simulink model "Rod_end_v7c"  (R2023a)
settings: Solver=ode1be  StartTime=0.0  StopTime=3  FixedStep=1e-6  MaxStep=1e-5  RelTol=1e-3
values from neighbouring files (symbols this model uses):
  A1_la = 5.710000e-003    (= 0.00571)    [C1_Actuator_1_Data.m]
  A2_la = 5.710000e-003    (= 0.00571)    [C1_Actuator_1_Data.m]
  a_jetpipe_area = 0    [B2_Main_file_Double_Active_Standby_System.m]
  A_svfb = 79.12.*1E-9.*sqrt(pi)    [B2_Main_file_Double_Active_Standby_System.m]
  a_svfb0_1 = 1E-3    (= 0.001)    [B2_Main_file_Double_Active_Standby_System.m]
  a_svfb0_2 = 0    [B2_Main_file_Double_Active_Standby_System.m]
  Afl_sv = dfl_sv^2*pi/4    (= 2.01519637574e-09)    [C1_Actuator_1_Data.m]
  Ag_sv = 18e-6    (= 1.8e-05)    [C1_Actuator_1_Data.m]
  air_gap0_1 = 0    [B2_Main_file_Double_Active_Standby_System.m]
  air_gap_fault_time = 10000    [B2_Main_file_Double_Active_Standby_System.m]
  Alpha_p0 = eta-acos((L^2+t^2-s^2)/(2*L*t))    [Parametri_rod_end.m]
  Asp_sv = 1.35e-5    (= 1.35e-05)    [C1_Actuator_1_Data.m]
  B0_sv = 0.460    (= 0.46)    [C1_Actuator_1_Data.m]
  b_airgap = 0.3    [B2_Main_file_Double_Active_Standby_System.m]
  b_fbspring = 2E-3    (= 0.002)    [B2_Main_file_Double_Active_Standby_System.m]
  b_max = 0*0.0001    (= 0)    [C1_Actuator_1_Data.m]
  beta = 800000000    [D4_Fluid.m]    (also in Rapporto_di_trasmissione.m = acos((L-t.*cos(alpha))./s))
  Beta0 = acos((L-t*cos(Alpha0))/s)    [Parametri_rod_end.m]
  beta_LVDT = 0    [aggiunte.m]
  bf_sv = 0.45    [C1_Actuator_1_Data.m]
  bsp_sv = 0.25    [C1_Actuator_1_Data.m]
  c = 55    [Parametri_rod_end.m]
  C_svfb = 1    [B2_Main_file_Double_Active_Standby_System.m]
  Cdmax_sv = 0.7392    [C1_Actuator_1_Data.m]
  Cdmin_sv = 0.6428    [C1_Actuator_1_Data.m]
  CLa = 900000    [aggiunte.m]
  Csa_la = 0.02*sqrt(Ksa_la*Meq_la)    [C1_Actuator_1_Data.m]
  Damping = 1e3    (= 1000)    [Parametri_rod_end.m]
  Damping_rot = 100    [Parametri_rod_end.m]
  Del_on = 1    [B2_Main_file_Double_Active_Standby_System.m]
  demag0_1 = 0    [B2_Main_file_Double_Active_Standby_System.m]
  dfl_sv = 5.0654e-5    (= 5.0654e-05)    [C1_Actuator_1_Data.m]
  dt_sim = 1e-5    (= 1e-05)    [B2_Main_file_Double_Active_Standby_System.m]
  enable_jetpipe_distorsion = 0    [B2_Main_file_Double_Active_Standby_System.m]
  eta = deg2rad(15)    [Parametri_rod_end.m]
  F_att_sv = 4    [C1_Actuator_1_Data.m]
  FH = FH+0.175*pi*Dd_se(ii)*(-0.884+0.0206*Hs_se(ii)-0.0001*(Hs_se(ii))^2)*Tw_se(ii)    [D2_Data_seal.m]
  first_cycle = 0    [B2_Main_file_Double_Active_Standby_System.m]
  flight_hours = 8    [B2_Main_file_Double_Active_Standby_System.m]
  g = 9.81    [Parametri_rod_end.m]
  g_sv = G_sv/l0_sv    (= 0)    [C1_Actuator_1_Data.m]
  Gamma_la = 1.667e4    (= 16670)    [C1_Actuator_1_Data.m]
  gap_ms = 0    [C1_Actuator_1_Data.m]
  Gq_sv = 0.069    [C1_Actuator_1_Data.m]
  Gust_stiffness_jetpipe = 1e8    (= 100000000)    [B2_Main_file_Double_Active_Standby_System.m]
  Gust_threshold = 10000    [B2_Main_file_Double_Active_Standby_System.m]
  h_fbspring = 1E-3    (= 0.001)    [B2_Main_file_Double_Active_Standby_System.m]
  h_sv = H_sv/l0_sv    (= 0)    [C1_Actuator_1_Data.m]
  hr_sv = 6e-6    (= 6e-06)    [C1_Actuator_1_Data.m]
  hyd_fluid_repl = 20    [B2_Main_file_Double_Active_Standby_System.m]
  I = 2.3    [Parametri_rod_end.m]    (also in Rapporto_di_trasmissione.m)
  imax_sv = 8e-3    (= 0.008)    [C1_Actuator_1_Data.m]
  Initial_condition = [0;0;0.000]    [Parametri_rod_end.m]
  Ixx_out = 0.0000321    (= 3.21e-05)    [Parametri_rod_end.m]
  Iyy_in = 0.0000008    (= 8e-07)    [Parametri_rod_end.m]
  Iyy_out = 0.0000035    (= 3.5e-06)    [Parametri_rod_end.m]
  Izz_in = 0.00000011    (= 1.1e-07)    [Parametri_rod_end.m]
  Izz_out = 0.0000337    (= 3.37e-05)    [Parametri_rod_end.m]
  Ja_sv = 1.0575e-5    (= 1.0575e-05)    [C1_Actuator_1_Data.m]
  jetpipe_initialpos = 0    [B2_Main_file_Double_Active_Standby_System.m]
  jetpipe_passage_area = 1    [B2_Main_file_Double_Active_Standby_System.m]
  k = 4/(3*pi*(sigma_j+sigma_k))*((R_in*R_out)/(R_in+R_out))^0.5    (= 15092124693.8)    [Parametri_rod_end.m]
  k_airgap = 0.5/100*0.01    (= 5e-05)    [B2_Main_file_Double_Active_Standby_System.m]
  k_c0_jetpipe_area = 0*1e-1    (= 0)    [B2_Main_file_Double_Active_Standby_System.m]
  k_sv = mup_sv*Vp_sv/(2*B0_sv*l0_sv)-1    (= 16.0383594613)    [C1_Actuator_1_Data.m]
  Kf_sv = 301.6    [C1_Actuator_1_Data.m]
  KFPi = zeros(m,1)    [D2_Data_seal.m]
  Kli1 = 0    [C1_Actuator_1_Data.m]
  Kli2 = 0    [C1_Actuator_1_Data.m]
  Ksa_la = 12480000    [C1_Actuator_1_Data.m]
  Kw_sv = 14.5    [C1_Actuator_1_Data.m]
  L = 0.37    [Parametri_rod_end.m]    (also in Rapporto_di_trasmissione.m = l+delta_l)
  l0_sv = 0.5e-3    (= 0.0005)    [C1_Actuator_1_Data.m]
  L_c = imax_sv    (= 0.008)    [C1_Actuator_1_Data.m]
  L_la1 = 0.059900    (= 0.0599)    [C1_Actuator_1_Data.m]
  L_la2 = 0.084800    (= 0.0848)    [C1_Actuator_1_Data.m]
  la_sv = 41e-3    (= 0.041)    [C1_Actuator_1_Data.m]
  lambda_LVDT = 0*0.005*1.5    (= 0)    [aggiunte.m]
  lf = 0.025    [C1_Actuator_1_Data.m]    (also in C2_Actuator_2_Data.m)
  LVDTsize0 = 1    [aggiunte.m]
  m_in = 0.0215    [Parametri_rod_end.m]
  m_out = 0.1    [Parametri_rod_end.m]
  m_thermal = 0    [B2_Main_file_Double_Active_Standby_System.m]
  Mcyl_la = 30.425550    (= 30.42555)    [C1_Actuator_1_Data.m]
  Mrod_la = 11.313490    (= 11.31349)    [C1_Actuator_1_Data.m]
  msp_sv = 0.005    [C1_Actuator_1_Data.m]
  mua_sv = 4*pi/1e7    (= 1.25663706144e-06)    [C1_Actuator_1_Data.m]
  mup_sv = 1.1*4*pi/1e7    (= 1.38230076758e-06)    [C1_Actuator_1_Data.m]
  n1_sv = 1140    [C1_Actuator_1_Data.m]
  n2_sv = 1140    [C1_Actuator_1_Data.m]
  n_svfb = 3    [B2_Main_file_Double_Active_Standby_System.m]
  null_shift = -1+2*rand(1,1)    [B2_Main_file_Double_Active_Standby_System.m]
  null_shift_sign = -1+((-1+2*rand(1,1))>=0)*2    [B2_Main_file_Double_Active_Standby_System.m]
  OV_R1 = 0*2.344e-05    (= 0)    [C1_Actuator_1_Data.m]
  OV_R2 = 0*2.344e-05    (= 0)    [C1_Actuator_1_Data.m]
  OV_S1 = 0*2.344e-05    (= 0)    [C1_Actuator_1_Data.m]
  OV_S2 = 0*2.344e-05    (= 0)    [C1_Actuator_1_Data.m]
  P01_la = Pmean-DP_eq    [C1_Actuator_1_Data.m]
  P02_la = Pmean+DP_eq    [C1_Actuator_1_Data.m]
  perc_passage_area0_1 = 0    [B2_Main_file_Double_Active_Standby_System.m]
  Pocl_A = 0    [C1_Actuator_1_Data.m]
  Pocl_B = 0    [C1_Actuator_1_Data.m]
  Pr = 600000    [B2_Main_file_Double_Active_Standby_System.m]
  Ps = 35000000    [B2_Main_file_Double_Active_Standby_System.m]
  R_in = 0.019    [Parametri_rod_end.m]
  R_out = 0.0195    [Parametri_rod_end.m]
  R_th1 = 0    [B2_Main_file_Double_Active_Standby_System.m]
  Remax_sv = 5000    [C1_Actuator_1_Data.m]
  Resistance = 1    [C1_Actuator_1_Data.m]
  rj_sv = 1e-6    (= 1e-06)    [C1_Actuator_1_Data.m]
  Rp02_svspring = 1014    [B2_Main_file_Double_Active_Standby_System.m]
  s = 0.11    [Parametri_rod_end.m]    (also in Rapporto_di_trasmissione.m)
  sigma_0LVDT = 0*0.01*1.5*5    (= 0)    [aggiunte.m]
  ST_AD = ceil(10000/fs_AD)/10000    [C1_Actuator_1_Data.m]
  Stiffness_rot = 1e3    (= 1000)    [Parametri_rod_end.m]
  Stifness = 1e8    (= 100000000)    [Parametri_rod_end.m]
  sv_crackON1 = 0    [B2_Main_file_Double_Active_Standby_System.m]
  sv_crackON2 = 0    [B2_Main_file_Double_Active_Standby_System.m]
  T0 = 0    [aggiunte.m]
  tau_w1 = 0    [B2_Main_file_Double_Active_Standby_System.m]
  ... (+14 more)
undefined symbols (not defined in the file or in its folder): Ixx_in, magnitude, mass, muu, Newton, R_sp_C, Raphson
libraries: simulink x16, matrix_library x12, sharedutil x2
(part 4 of 4)

== system Rod_end_v7c/Attuatore/Actuation System/Servovalve/Spool/orifice2S-resistences/Cd ==
  In2 : Inport
  In1 : Inport  Port=2
  In3 : Inport  Port=3
  Abs : Abs  SaturateOnIntegerOverflow=off
  Fcn : Fcn  Expr=0.22*sqrt(log(1+u(1)))
  Fcn1 : Fcn  Expr=u(2)*(1+0.2*hr_sv/(u(1)+hr_sv))
  Fcn2 : Fcn  Expr=2*u(3)*u(2)/(u(4)*(wsp_sv+u(1)))
  Fcn3 : Fcn  Expr=(u(2)*(u(1)+u(3)))/(2*(u(1)*u(3)))
  Lookup Table1 : Lookup  InputValues=R_sp_C(1,:)  Table=R_sp_C(2,:)  SaturateOnIntegerOverflow=off
  Memory1 : Memory  InitialCondition=eps
  Mux1 : Mux  Inputs=2
  Mux2 : Mux  Inputs=3
  Mux3 : Mux  Inputs=3
  Product : Product  RndMeth=Zero
  Saturation : Saturate  UpperLimit=Remax_sv  LowerLimit=0
  Saturation1 : Saturate  UpperLimit=Cdmax_sv  LowerLimit=Cdmin_sv
  Scope2 : Scope  NumInputPorts=2
  gioco radiale2 : Constant  Value=rj_sv
  gioco radiale3 : Constant  Value=wsp_sv
  Out3 : Outport
  wires:
  Fcn2/1 -> Saturation/1
  Saturation/1 -> Fcn/1
  Fcn/1 -> Mux1/2  "Cd0"
  Mux1/1 -> Fcn1/1
  Fcn1/1 -> Saturation1/1  "Cd"
  In3/1 -> Mux2/1, Mux3/1  "l[m]"
  Memory1/1 -> Mux2/2
  In2/1 -> Memory1/1  "Q1R[m3/s]"
  Mux2/1 -> Fcn2/1
  In1/1 -> Abs/1  "x[m]"
  gioco radiale3/1 -> Mux3/3
  Lookup Table1/1 -> Product/2  "c'"
  Mux3/1 -> Fcn3/1
  gioco radiale2/1 -> Mux3/2
  Fcn3/1 -> Lookup Table1/1  "r/d0"
  Product/1 -> Scope2/2, Out3/1  "Cd"
  Saturation1/1 -> Product/1, Scope2/1  "Cd"
  Abs/1 -> Mux1/1
  [Fluid_properties_var] -> Mux2/3

== system Rod_end_v7c/Attuatore/Actuation System/Servovalve/Servovalve Dynamic/Jet pipe dynamic/Double Integrator/Limit ==
  In2 : Inport
  In1 : Inport  Port=2
  Constant : Constant
  Constant1 : Constant  Value=-1
  Constant2 : Constant  Value=0
  Constant3 : Constant  Value=0
  Logical Operator : Logic  AllPortsSameDT=off
  Logical Operator1 : Logic  AllPortsSameDT=off
  Logical Operator2 : Logic  Operator=NOR  AllPortsSameDT=off
  Product : Product  RndMeth=Zero
  Relational Operator : RelationalOperator  Operator=>  OutDataTypeStr=boolean  InputSameDT=off
  Relational Operator1 : RelationalOperator  Operator===  OutDataTypeStr=boolean  InputSameDT=off
  Relational Operator2 : RelationalOperator  Operator=<  OutDataTypeStr=boolean  InputSameDT=off
  Relational Operator3 : RelationalOperator  Operator===  OutDataTypeStr=boolean  InputSameDT=off
  Out2 : Outport
  wires:
  In2/1 -> Relational Operator/1, Product/1, Relational Operator2/1  "xrod_dd [m/s2]"
  In1/1 -> Relational Operator3/1, Relational Operator1/1  "limit xrod"
  Constant3/1 -> Relational Operator/2
  Constant/1 -> Relational Operator1/2
  Constant1/1 -> Relational Operator3/2
  Constant2/1 -> Relational Operator2/2
  Relational Operator/1 -> Logical Operator/1
  Relational Operator1/1 -> Logical Operator/2
  Relational Operator3/1 -> Logical Operator1/1
  Relational Operator2/1 -> Logical Operator1/2
  Logical Operator/1 -> Logical Operator2/1
  Logical Operator1/1 -> Logical Operator2/2
  Logical Operator2/1 -> Product/2
  Product/1 -> Out2/1  "xrod_dd [m2/s]"

== system Rod_end_v7c/Attuatore/Actuation System/Servovalve/Servovalve Dynamic/Spool  dynamic/Double Integrator/Limit ==
  In2 : Inport
  In1 : Inport  Port=2
  Constant : Constant
  Constant1 : Constant  Value=-1
  Constant2 : Constant  Value=0
  Constant3 : Constant  Value=0
  Logical Operator : Logic  AllPortsSameDT=off
  Logical Operator1 : Logic  AllPortsSameDT=off
  Logical Operator2 : Logic  Operator=NOR  AllPortsSameDT=off
  Product : Product  RndMeth=Zero
  Relational Operator : RelationalOperator  Operator=>  OutDataTypeStr=boolean  InputSameDT=off
  Relational Operator1 : RelationalOperator  Operator===  OutDataTypeStr=boolean  InputSameDT=off
  Relational Operator2 : RelationalOperator  Operator=<  OutDataTypeStr=boolean  InputSameDT=off
  Relational Operator3 : RelationalOperator  Operator===  OutDataTypeStr=boolean  InputSameDT=off
  Out2 : Outport
  wires:
  In2/1 -> Relational Operator/1, Product/1, Relational Operator2/1  "xrod_dd [m/s2]"
  In1/1 -> Relational Operator3/1, Relational Operator1/1  "limit xrod"
  Constant3/1 -> Relational Operator/2
  Constant/1 -> Relational Operator1/2
  Constant1/1 -> Relational Operator3/2
  Constant2/1 -> Relational Operator2/2
  Relational Operator/1 -> Logical Operator/1
  Relational Operator1/1 -> Logical Operator/2
  Relational Operator3/1 -> Logical Operator1/1
  Relational Operator2/1 -> Logical Operator1/2
  Logical Operator/1 -> Logical Operator2/1
  Logical Operator1/1 -> Logical Operator2/2
  Logical Operator2/1 -> Product/2
  Product/1 -> Out2/1  "xrod_dd [m2/s]"

== system Rod_end_v7c/Attuatore/Actuation System/Servovalve/Servovalve Dynamic/Spool  dynamic/Flow Force/Q_max evaluation and flow angle variation ==
  In1 : Inport
  In2 : Inport  Port=2
  In3 : Inport  Port=3
  Constant3 : Constant  Value=Cdmin_sv
  Product3 : Product
  Product4 : Product
  Total Passage Area : Subsystem
  Variation of flow angle Q1 : Subsystem
  Variation of flow angle Q2 : Subsystem
  sqrt(0.5*dP/ro) : Fcn  Expr=sqrt(0.5*(u(1)-u(2))/u(3))
  cos(teta) of Q1 : Outport
  cos(teta) of Q2 : Outport  Port=2
  wires:
  Constant3/1 -> Product3/2
  sqrt(0.5*dP/ro)/1 -> Product4/1
  Total Passage Area/1(Out3) -> Product3/1
  Product3/1 -> Product4/2
  Product4/1 -> Variation of flow angle Q1/2(In3), Variation of flow angle Q2/1(In3)  "Q_max [m3/s]"
  Variation of flow angle Q1/1(cos(teta)) -> cos(teta) of Q1/1
  In1/1 -> Variation of flow angle Q1/1(In1)
  Variation of flow angle Q2/1(cos(teta)) -> cos(teta) of Q2/1
  In2/1 -> sqrt(0.5*dP/ro)/1
  In3/1 -> Variation of flow angle Q2/2(In1)

== system Rod_end_v7c/Attuatore/Actuation System/Servovalve/Servovalve Dynamic/Torque Motor/air gap evaluation/Activation conditions ==
  Add1 : Sum  Inputs=+|-
  Add2 : Sum  Inputs=+|+
  Clock : Clock
  Compare To Constant : simulink/Logic and Bit Operations/Compare To Constant  relop=>  const=0  OutDataTypeStr=uint8
  Constant1 : Constant  Value=air_gap_fault_time
  Constant2 : Constant  Value=first_cycle-1
  Constant3 : Constant  Value=flight_hours
  Gain1 : Gain  Gain=flight_hours/364
  Product1 : Product  SaturateOnIntegerOverflow=on  OutDataTypeStr=Inherit: Same as first input
  Product2 : Product  SaturateOnIntegerOverflow=on  OutDataTypeStr=Inherit: Same as first input
  Relational Operator : RelationalOperator  Operator=<  OutDataTypeStr=boolean  InputSameDT=off
  Saturation : Saturate  UpperLimit=inf  LowerLimit=0
  Out2 : Outport
  Out1 : Outport  Port=2
  tag scope: flight_time=global
  wires:
  Constant2/1 -> Saturation/1
  Constant3/1 -> Product2/2
  Product2/1 -> Add2/1
  Clock/1 -> Gain1/1
  Gain1/1 -> Add2/2
  Constant1/1 -> Relational Operator/1, Add1/2
  Add2/1 -> Relational Operator/2, Add1/1, [flight_time]  "flight time [h]"
  Relational Operator/1 -> Out1/1  "enable_com"
  Add1/1 -> Compare To Constant/1, Product1/1
  Compare To Constant/1 -> Product1/2
  Product1/1 -> Out2/1  "flight time [h]"
  Saturation/1 -> Product2/1

== system Rod_end_v7c/Attuatore/Actuation System/Servovalve/Servovalve Dynamic/Torque Motor/air gap evaluation/counter ==
  In1 : Inport
  Enable : EnablePort
  Add2 : Sum  Inputs=+|+
  Compare To Constant : simulink/Logic and Bit Operations/Compare To Constant  relop=>  const=0  OutDataTypeStr=uint8
  Data Type Conversion1 : DataTypeConversion  OutDataTypeStr=double  SaturateOnIntegerOverflow=off  RndMeth=Floor
  Memory : Memory
  Out1 : Outport
  wires:
  Add2/1 -> Memory/1, Out1/1
  Compare To Constant/1 -> Data Type Conversion1/1
  In1/1 -> Compare To Constant/1
  Memory/1 -> Add2/2
  Data Type Conversion1/1 -> Add2/1

== system Rod_end_v7c/Attuatore/Actuation System/Servovalve/Servovalve Dynamic/Spool  dynamic/Flow Force/Q_max evaluation and flow angle variation/Total Passage Area ==
  note: Xvr1 +Xvr2
  note: Xvs1 +Xvs2
  Add1 : Sum  Inputs=-|+
  Add2 : Sum  Inputs=+|-
  Add3 : Sum  Inputs=-|+
  Add4 : Sum  Inputs=+|-
  Add5 : Sum  Inputs=+|+
  Add6 : Sum  Inputs=+|+
  Add7 : Sum  Inputs=+|+
  Constant3 : Constant  Value=xspmax_sv
  Gain : Gain  Gain=0.5
  MinMax{,1..3} (4 alike) : MinMax  Inputs=2
  Product : Product
  Product1 : Product
  gioco radiale1 : Constant  Value=wsp_sv
  ricoprimento : Constant  Value=OV_S1
  ricoprimento1 : Constant  Value=OV_S2
  ricoprimento2 : Constant  Value=OV_R1
  ricoprimento3 : Constant  Value=OV_R2
  Out3 : Outport
  wires:
  ricoprimento/1 -> Add3/1
  Constant3/1 -> Add2/1, Add1/2, Add3/2, MinMax1/2, MinMax/1, Add4/1, MinMax3/1, MinMax2/2
  ricoprimento1/1 -> Add1/1
  ricoprimento2/1 -> Add2/2
  ricoprimento3/1 -> Add4/2
  Add6/1 -> Product/1
  gioco radiale1/1 -> Product1/1, Product/2
  Add5/1 -> Product1/2
  Product1/1 -> Add7/2  "A_VR"
  Product/1 -> Add7/1  "A_VS"
  Add7/1 -> Gain/1
  Gain/1 -> Out3/1  "A_median"
  Add1/1 -> MinMax/2
  Add3/1 -> MinMax1/1
  MinMax/1 -> Add6/2
  MinMax1/1 -> Add6/1
  Add4/1 -> MinMax3/2
  Add2/1 -> MinMax2/1
  MinMax2/1 -> Add5/1
  MinMax3/1 -> Add5/2

== system Rod_end_v7c/Attuatore/Actuation System/Servovalve/Servovalve Dynamic/Spool  dynamic/Flow Force/Q_max evaluation and flow angle variation/Variation of flow angle Q1 ==
  In1 : Inport
  In3 : Inport  Port=2
  Constant4 : Constant  Value=0.5
  Flow less than 0.05 : Fcn  Expr=1-10*u(1)
  Product5 : Product  Inputs=*/  SaturateOnIntegerOverflow=on  OutDataTypeStr=Inherit: Same as first input
  Switch : Switch  Criteria=u2 > Threshold  Threshold=0.05  SaturateOnIntegerOverflow=off  InputSameDT=off
  cos(teta) : Outport
  wires:
  Switch/1 -> cos(teta)/1
  Constant4/1 -> Switch/1
  Product5/1 -> Flow less than 0.05/1, Switch/2
  In1/1 -> Product5/1
  In3/1 -> Product5/2
  Flow less than 0.05/1 -> Switch/3

== system Rod_end_v7c/Attuatore/Actuation System/Servovalve/Servovalve Dynamic/Spool  dynamic/Flow Force/Q_max evaluation and flow angle variation/Variation of flow angle Q2 ==
  In3 : Inport
  In1 : Inport  Port=2
  Constant4 : Constant  Value=0.5
  Flow less than 0.05 : Fcn  Expr=1-10*u(1)
  Product5 : Product  Inputs=*/  SaturateOnIntegerOverflow=on  OutDataTypeStr=Inherit: Same as first input
  Switch : Switch  Criteria=u2 > Threshold  Threshold=0.05  SaturateOnIntegerOverflow=off  InputSameDT=off
  cos(teta) : Outport
  wires:
  Switch/1 -> cos(teta)/1
  Constant4/1 -> Switch/1
  Product5/1 -> Flow less than 0.05/1, Switch/2
  In1/1 -> Product5/1
  In3/1 -> Product5/2
  Flow less than 0.05/1 -> Switch/3
